simulink model "PID"  (R2023b)
settings: Solver=ode8  StartTime=0.0  StopTime=20  FixedStep=0.005  RelTol=1e-3
settings Model: Creator=suvo  LastModifiedBy=suvo
settings SolverCC: AlgebraicLoopSolver=TrustRegion
settings DataIOCC: ReturnWorkspaceOutputs=off
settings DebuggingCC: UnconnectedInputMsg=warning  UnconnectedOutputMsg=warning  UnconnectedLineMsg=warning
settings ModelReferenceCC: EnableRefExpFcnMdlSchedulingChecks=on

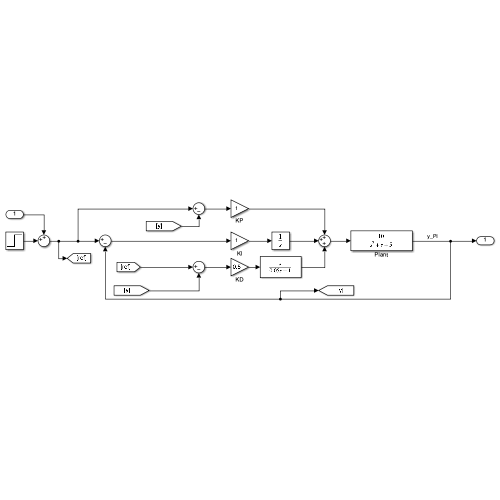
[thumbnail: Simulink's stored preview of the top-level diagram]
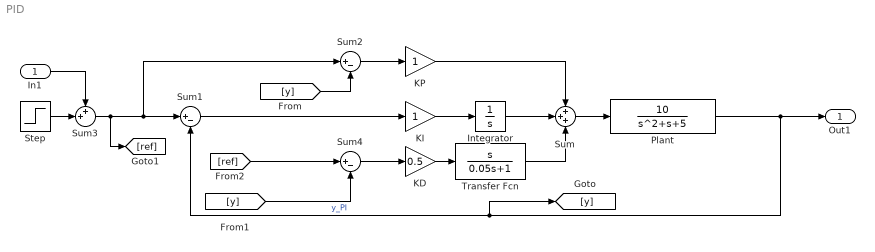
== system PID ==
  In1 : Inport
  Integrator : Integrator
  KD : Gain  Gain=0.5
  KI : Gain
  KP : Gain
  Plant : TransferFcn  Numerator=10  Denominator=[1 1 5]
  Step : Step  SampleTime=0
  Sum : Sum  Inputs=+++
  Sum1 : Sum  Inputs=|+-
  Sum2 : Sum  Inputs=|+-
  Sum3 : Sum  Inputs=++|
  Sum4 : Sum  Inputs=|+-
  Transfer Fcn : TransferFcn  Numerator=[1 0]  Denominator=[0.05 1]
  Out1 : Outport
  wires:
  KI/1 -> Integrator/1
  Sum1/1 -> KI/1
  Plant/1 -> [y], Sum1/2, Out1/1  "y_PI"
  Sum2/1 -> KP/1
  KP/1 -> Sum/1
  Integrator/1 -> Sum/2
  Sum/1 -> Plant/1
  In1/1 -> Sum3/1
  Step/1 -> Sum3/2
  [y] -> Sum2/2
  KD/1 -> Transfer Fcn/1
  Transfer Fcn/1 -> Sum/3
  Sum4/1 -> KD/1
  [y] -> Sum4/2
  [ref] -> Sum4/1
  Sum3/1 -> Sum2/1, Sum1/1, [ref]
